simulink model "implementation"  (R2014b)
settings: Solver=ode45  StartTime=0.0  StopTime=4  RelTol=1e-3
values from neighbouring files (symbols this model uses):
  DEN = DEN{1}(2:end)    [print_control.m]
  dv = 1e-5    (= 1e-05)    [DCparamsPD.m]    (also in DCparamsPI.m; DCparamsPID.m)
  eta = 0.74    [DCparamsPD.m]    (also in DCparamsPI.m = 0.75; DCparamsPID.m = 0.75)
  J = 0.05    [DCparamsPD.m]    (also in DCparamsPI.m; DCparamsPID.m; beam_friction.m = 0.000914666666667)
  K = 0.0229    [DCparamsPD.m]    (also in DCparamsPI.m = 0.0214; DCparamsPID.m = 0.0214)
  k_f = [0.072091, 0.040963, -0.003493]    [DCparamsPD.m]    (also in DCparamsPI.m; DCparamsPID.m)
  L = 0.192e-3    (= 0.000192)    [DCparamsPD.m]    (also in DCparamsPI.m = 0.000129; DCparamsPID.m = 0.000129; beam_friction.m = 0.2)
  n = 300564.0/1300.0    (= 231.203076923)    [DCparamsPD.m]    (also in DCparamsPI.m = 149.526172053; DCparamsPID.m = 149.526172053; print_control.m = %0.4f)
  NUMfb = NUMfb{1}    [print_control.m]
  NUMff = NUMff{1}    [print_control.m]
  R = 1.83 + 0.33    (= 2.16)    [DCparamsPD.m]    (also in DCparamsPI.m = 1.07; DCparamsPID.m = 1.07; furuta_controller.m = 10; ik_test.m = 0.15925)
  Ts = 1 / 320    (= 0.003125)    [DCparamsPD.m]    (also in DCparamsPI.m = 0.002; DCparamsPID.m = 0.0016; ik_test.m = 0.0333333333333; read_log_file.m = mean(diff(D{end}.time)))
libraries: cstblocks x2, simulink x1
settings Model: Creator=vkozma  LastModifiedBy=vkozma

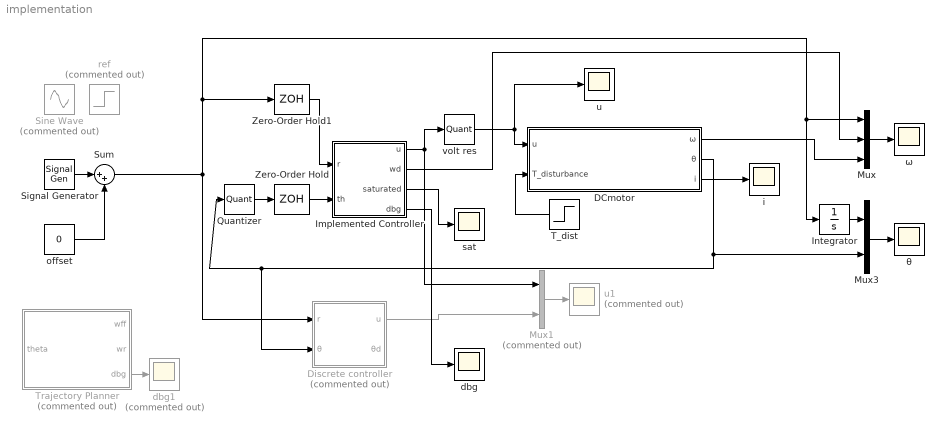
== system implementation ==
  DCmotor : Subsystem
  Discrete controller : Subsystem  Commented=on
  Implemented Controller : MATLAB Function  TreatAsAtomicUnit=on
  Integrator : Integrator
  Mux : Mux  Inputs=3
  Mux1 : Mux  Commented=on  Inputs=2
  Mux3 : Mux  Inputs=2
  Quantizer : Quantizer  QuantizationInterval=enc_res
  Signal Generator : SignalGenerator  WaveForm=square  Amplitude=2
  Sine Wave : Sin  Commented=on  Amplitude=2  Frequency=2*pi/4  SampleTime=0
  Sum : Sum  Inputs=|++
  T_dist : Step  Time=2  After=0  SampleTime=0
  Trajectory Planner : MATLAB Function  Commented=on  TreatAsAtomicUnit=on
  Zero-Order Hold : ZeroOrderHold  SampleTime=Ts
  Zero-Order Hold1 : ZeroOrderHold  SampleTime=Ts
  dbg : Scope
      settings: SaveName=ScopeData9
  dbg1 : Scope  Commented=on
      settings: TimeRange=0.1147540983606558  YMin=-1  YMax=1  SaveName=ScopeData10
  i : Scope
      settings: SaveName=ScopeData2
  offset : Constant  Value=0
  ref : Step  Commented=on  Time=0  After=-2  SampleTime=0
  sat : Scope
      settings: SaveName=ScopeData4
  u : Scope
  u1 : Scope  Commented=on
      settings: SaveName=ScopeData3
  volt res : Quantizer  QuantizationInterval=volt_res
  θ : Scope
      settings: SaveName=ScopeData6
  ω : Scope
  wires:
  DCmotor/1(ω) -> Mux/3
  Mux/1 -> ω/1
  Implemented Controller/1(u) -> Mux1/1, volt res/1
  DCmotor/2(θ) -> Mux3/2, Discrete controller/2(θ), Quantizer/1
  Implemented Controller/2(wd) -> Mux/2
  DCmotor/3(i) -> i/1
  T_dist/1 -> DCmotor/2(T_disturbance)
  Quantizer/1 -> Zero-Order Hold/1
  Zero-Order Hold/1 -> Implemented Controller/2(th)
  Zero-Order Hold1/1 -> Implemented Controller/1(r)
  Mux1/1 -> u1/1
  Discrete controller/1(u) -> Mux1/2
  Mux3/1 -> θ/1
  Implemented Controller/3(saturated) -> sat/1
  Implemented Controller/4(dbg) -> dbg/1
  Signal Generator/1 -> Sum/1
  offset/1 -> Sum/2
  Integrator/1 -> Mux3/1
  Sum/1 -> Zero-Order Hold1/1, Mux/1, Integrator/1, Discrete controller/1(r)
  volt res/1 -> DCmotor/1(u), u/1
  Trajectory Planner/3(dbg) -> dbg1/1

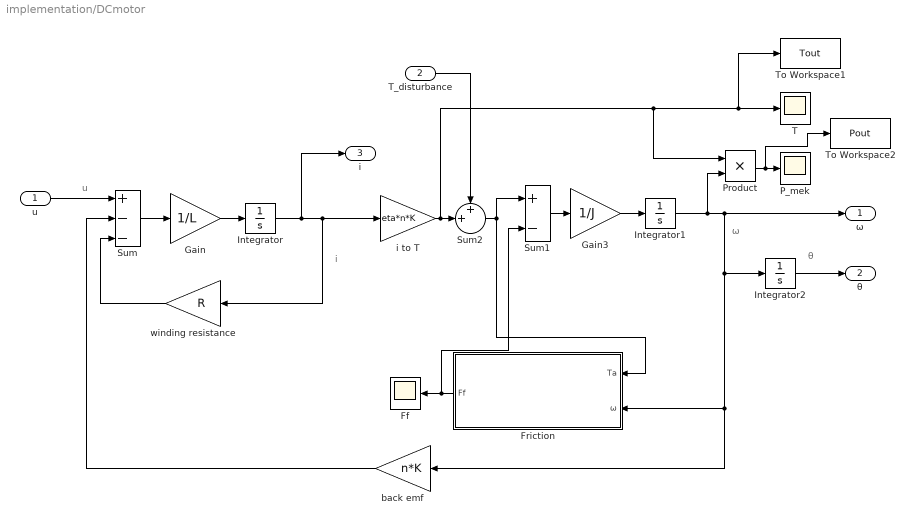
== system implementation/DCmotor ==
  note: θ
  note: ω
  note: i
  note: u
  u : Inport
  T_disturbance : Inport  Port=2
  Ff : Scope
      settings: SaveName=ScopeData5
  Friction : Subsystem
  Gain : Gain  Gain=1/L
  Gain3 : Gain  Gain=1/J
  Integrator : Integrator
  Integrator1 : Integrator
  Integrator2 : Integrator
  P_mek : Scope
      settings: SaveName=ScopeData8
  Product : Product
  Sum : Sum  Inputs=+--
  Sum1 : Sum  Inputs=+-
  Sum2 : Sum  Inputs=++|
  T : Scope
      settings: SaveName=ScopeData7
  To Workspace1 : ToWorkspace  VariableName=Tout  SampleTime=1/100
      settings: Save2DSignal=2-D array (concatenate along first dimension)
  To Workspace2 : ToWorkspace  VariableName=Pout  SampleTime=1/100
      settings: Save2DSignal=2-D array (concatenate along first dimension)
  back emf : Gain  Gain=n*K
  i to T : Gain  Gain=eta*n*K
  winding resistance : Gain  Gain=R
  ω : Outport
  θ : Outport  Port=2
  i : Outport  Port=3
  wires:
  u/1 -> Sum/1
  Sum/1 -> Gain/1
  Gain/1 -> Integrator/1
  Integrator/1 -> i/1, winding resistance/1, i to T/1
  winding resistance/1 -> Sum/3
  Sum1/1 -> Gain3/1
  Gain3/1 -> Integrator1/1
  Integrator1/1 -> Product/2, ω/1, Integrator2/1, Friction/2(ω), back emf/1
  i to T/1 -> Sum2/2, Product/1, To Workspace1/1, T/1
  back emf/1 -> Sum/2
  Integrator2/1 -> θ/1
  Product/1 -> To Workspace2/1, P_mek/1
  Friction/1(Ff) -> Sum1/2, Ff/1
  Sum2/1 -> Friction/1(Ta), Sum1/1
  T_disturbance/1 -> Sum2/1

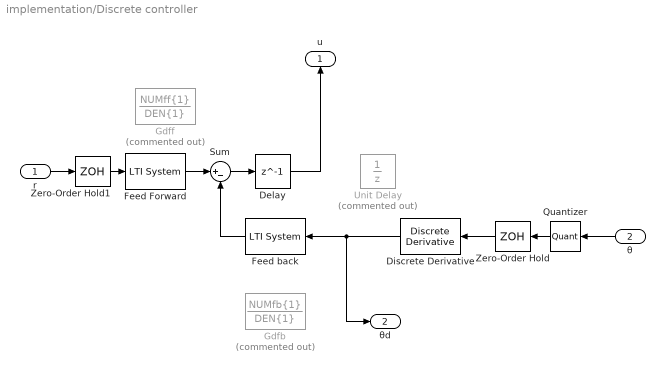
== system implementation/Discrete controller ==
  r : Inport
  θ : Inport  Port=2
  Delay : Delay  DelayLength=1
  Discrete Derivative : simulink/Discrete/Discrete Derivative  gainval=1.0  ICPrevScaledInput=0.0  InputProcessing=Inherited  OutMin=[]  OutMax=[]  OutDataType=fixdt(1, 16)  OutScaling=2^-10  DoSatur=off
  Feed Forward : cstblocks/LTI System  sys=Gdff  IC=[]
  Feed back : cstblocks/LTI System  sys=Gdfb  IC=[]
  Gdfb : DiscreteTransferFcn  Commented=on  Numerator=NUMfb{1}  Denominator=DEN{1}
  Gdff : DiscreteTransferFcn  Commented=on  Numerator=NUMff{1}  Denominator=DEN{1}
  Quantizer : Quantizer  QuantizationInterval=enc_res
  Sum : Sum  Inputs=|+-
  Unit Delay : UnitDelay  Commented=on  SampleTime=-1
  Zero-Order Hold : ZeroOrderHold  SampleTime=Ts
  Zero-Order Hold1 : ZeroOrderHold  SampleTime=Ts
  u : Outport
  θd : Outport  Port=2
  wires:
  r/1 -> Zero-Order Hold1/1
  θ/1 -> Quantizer/1
  Quantizer/1 -> Zero-Order Hold/1
  Zero-Order Hold/1 -> Discrete Derivative/1
  Sum/1 -> Delay/1
  Discrete Derivative/1 -> Feed back/1, θd/1
  Zero-Order Hold1/1 -> Feed Forward/1
  Delay/1 -> u/1
  Feed back/1 -> Sum/2
  Feed Forward/1 -> Sum/1

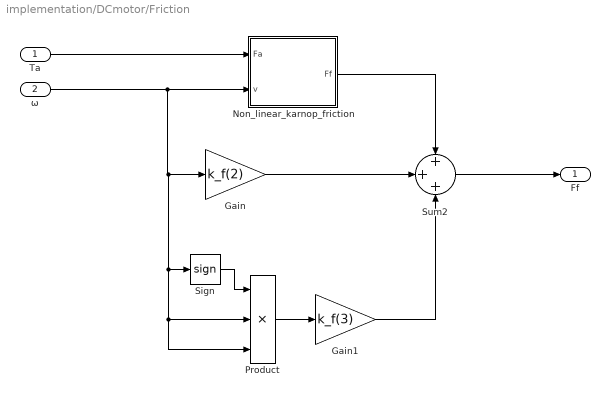
== system implementation/DCmotor/Friction ==
  Ta : Inport
  ω : Inport  Port=2
  Gain : Gain  Gain=k_f(2)
  Gain1 : Gain  Gain=k_f(3)
  Non_linear_karnop_friction : Subsystem
  Product : Product  Inputs=3
  Sign : Signum
  Sum2 : Sum  Inputs=+++
  Ff : Outport
  wires:
  ω/1 -> Product/3, Product/2, Sign/1, Gain/1, Non_linear_karnop_friction/2(v)
  Ta/1 -> Non_linear_karnop_friction/1(Fa)
  Sum2/1 -> Ff/1
  Non_linear_karnop_friction/1(Ff) -> Sum2/1
  Gain/1 -> Sum2/2
  Sign/1 -> Product/1
  Product/1 -> Gain1/1
  Gain1/1 -> Sum2/3

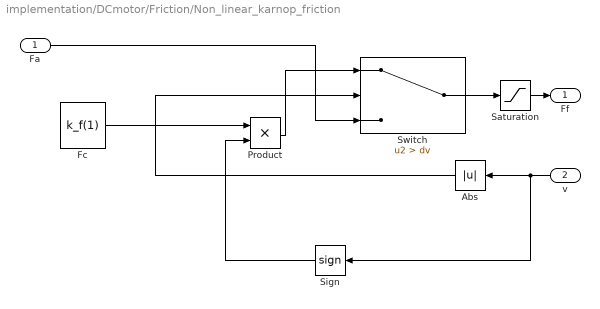
== system implementation/DCmotor/Friction/Non_linear_karnop_friction ==
  Fa : Inport
  v : Inport  Port=2
  Abs : Abs
  Fc : Constant  Value=k_f(1)
  Product : Product  RndMeth=Zero
  Saturation : Saturate  UpperLimit=k_f(1)  LowerLimit=-k_f(1)
  Sign : Signum
  Switch : Switch  Criteria=u2 > Threshold  Threshold=dv
  Ff : Outport
  wires:
  Sign/1 -> Product/2
  Fc/1 -> Product/1
  Abs/1 -> Switch/2
  Fa/1 -> Switch/3
  v/1 -> Abs/1, Sign/1
  Switch/1 -> Saturation/1
  Saturation/1 -> Ff/1
  Product/1 -> Switch/1

== matlab function implementation/Trajectory Planner ==
  data: wff output; theta input; wr output; dbg output
function [wff,wr,dbg] = fcn(theta)
% Trajectory planning for a speed controller
persistent theta_goal w_ff state theta_tot T_on prev_err cum_err dbg_val
persistent w_acc w_trans Ts P I D % Constants
if isempty(w_ff) % init traj planner
    % Inputs and stuff that may change
    theta_goal = 3;
    w_ff = 0;
    state = 3; % 0 = acc to w_trans, 1 = steady speed, 2 = decelerate to 0, 3 = keep at 0
    theta_tot = 0;
    T_on = 0; % timer
    prev_err = 0; cum_err = 0; % Feedback control
    dbg_val = 1;
    % Constants
    w_acc = 5; % rad/s/s
    w_trans = 1.8377; % rad/s
    Ts = 1/500; % Sample time
    P = 12.925; I = 37.0; D = 0.3; % PID-constants 
end % init

%%%%%%%%%%%%%%%%%%%%%%%%%% MASTER UNIT %%%%%%%%%%%%%%%%%%%%%%%%%%%%%%%%%

% Master unit, for issuing commands
persistent Ts_master prev_time pressed
if isempty(Ts_master) % init master
    Ts_master = 1/50;
    prev_time = 0;
    pressed = 0;
end
% Master loop
if (T_on - prev_time >= Ts_master)
    if pressed == 0 && T_on >= 2.5
        pressed = 1;
        theta_goal = 4;
        w_trans = 3.618033;
    end
    
    prev_time = T_on;%prev_time + Ts_master;
end

%%%%%%%%%%%%%%%%%%%%%% TRAJECTORY PLANNER %%%%%%%%%%%%%%%%%%%%%%%%%%%%%

% Check whether to start to break 
if (state < 2) && (abs(theta_goal - theta_tot) < w_ff*w_ff/(2*w_acc))
    state = 2;
end

switch state
    case 0 % acc to w_trans
        new_w = w_ff + sign(sign(theta_goal+eps)*w_trans - w_ff)*Ts*w_acc;
        if sign(new_w - sign(theta_goal+eps)*w_trans + eps) ~= sign(w_ff - sign(theta_goal+eps)*w_trans + eps)
            w_ff = sign(theta_goal+eps)*w_trans;
            state = 1;
        else
            w_ff = new_w;
        end
        
    case 1 % steady speed
        if abs(w_ff - sign(theta_goal+eps)*w_trans) > 1e-6 % new speed found
            state = 0;
        else
            w_ff = sign(theta_goal+eps)*w_trans;
        end
    case 2 % decelerate to zero speed
        new_w = w_ff - sign(w_ff+eps)*Ts*w_acc;
        if sign(new_w) ~= sign(w_ff)
            w_ff = 0;
            state = 3;
        else
            w_ff = new_w;
        end
    case 3 % stay at zero, at target
        w_ff = 0;
        if abs(theta_tot - theta_goal) < 1e-2
            theta_tot = theta_goal;
        end
        if abs(theta_tot - theta_goal) > 1e-3;
            state = 0;
            fprintf('t = %f, theta_tot = %f, theta_goal = %f\n',T_on,theta_tot,theta_goal);
        end
end

% feedback PID-control
err = theta_tot - theta;
w_fb = P*err + I*cum_err + D*(err - prev_err)/Ts;
prev_err = err;
cum_err = cum_err + err*Ts;

% Output 
wr = w_ff + w_fb;
wff = w_ff;

% debugging var
dbg = dbg_val;

% Update theta_tot
theta_tot = theta_tot + Ts * w_ff;
T_on = T_on + Ts;
end

== matlab function implementation/Implemented Controller ==
  data: r input; th input; u output; wd output; saturated output; dbg output
function [u,wd,saturated,dbg] = fcn(r,th)
persistent uout old_y old_r old_uff old_ufb prev_th I_ff I_fb old_spd issat
persistent cMode Ts nd d nc c nf f Id umax imax K R n% Constants
if isempty(uout) % init
    uout = 0; issat = 0;
    old_y = zeros(1,4); old_r = zeros(1,4);
    old_uff = zeros(1,4); old_ufb = zeros(1,4);
    prev_th = 0; I_ff = 0; I_fb = 0;
    old_spd = 0;
    % Generated constants from script, replace if new params
K = 0.0214; n = 149.5262; R = 1.0700;
cMode = 1; umax = 24.0; imax = 2.0;
Ts = 1/500.00;
nd = 2; d = [0.02358463,0.02358463];
nc = 2; c = [-0.62039556,0.88517879];
nf = 1; f = [-0.68842077];
Id = 0.20189841;
end % of init
u = uout;

if cMode == 0
    old_y(1) = th; %wd = (th - prev_th)/Ts; % Position control
else
    old_y(1) = (th - prev_th)/Ts; %wd = old_y(1); % Speed control
end
old_r(1) = r;

% ufb = d(2)*old_y(1) + d(1)*old_y(2) - f(2)*old_ufb(1) - f(1)*old_ufb(2);
% uff = c(3)*old_r(1) + c(2)*old_r(2) + c(1)*old_r(3) - f(2)*old_uff(1) - f(1)*old_uff(2);
ufb = 0; uff = 0;
for i = 1:nd
    ufb = ufb + d(i)*old_y(nd-i+1);
end
for i = 1:nc
    uff = uff + c(i)*old_r(nc-i+1);
end
for i = 1:nf
    ufb = ufb - f(i)*old_ufb(nf-i+1);
    uff = uff - f(i)*old_uff(nf-i+1);
end

% Integrators
skipping = 0.99;
%T_backcalc = 0.05;
if Id > 0 && issat == 0
%if Id > 0 && issat == 0 && (old_r(1) - old_y(1))*u_nosat >= 0
%if Id > 0 && issat == 0 && (I_ff - I_fb)*u_nosat >= 0
%if Id > 0
%     I_ff = I_ff + (Id + Ts*(uout - u_nosat)/T_backcalc)*old_r(1);
%     I_fb = I_fb + (Id - Ts*(uout - u_nosat)/T_backcalc)*old_y(1);
    I_ff = I_ff + Id*old_r(1);
    I_fb = I_fb + Id*old_y(1);
    skipping = 0.01;
end

% if Id > 0 % Skip if no integrator term is present
%     toupdate = 1;
%     if issat == 1 % if saturated don't update the terms
%         if sign(I_ff - I_fb) ~= sign(u_nosat) % if can't reach
%             toupdate = 0;
%         end
%         toupdate = 0;
%     end
%     if toupdate == 1
%         I_ff = I_ff + Id*old_r(1);
%         I_fb = I_fb + Id*old_y(1);
%         skipping = 0.01; % debug variable
%     end
% end


saturated = 0.98*issat + 0.01; % test

uout = (uff + I_ff) - (ufb + I_fb);

% Current and voltage limiting
issat = 0; u_nosat = uout;
% voltage limiting
if uout > umax
    uout = umax;
    issat = 1;
elseif uout < -umax
    uout = -umax;
    issat = 1;
end

% current limiting
%if Id == 0 % Anti windup may get wonky with the current limiter
    curr_lim_dlpfc = 0.2;
    spd = (th - prev_th)/Ts;
    spd = curr_lim_dlpfc*spd + (1 - curr_lim_dlpfc)*old_spd;
    old_spd = spd;
    temp1 = K*n*spd; temp2 = R*imax;
    if uout > (temp1 + temp2), 
        uout = temp1 + temp2; 
        issat = 1;
    elseif uout < (temp1 - temp2) 
        uout = temp1 - temp2; 
        issat = 1;
    end
%end

% Debugging output
wd = (th - prev_th)/Ts; 
dbg = [skipping,saturated];%, 1.01*sign(I_ff - I_fb), 0.95*sign(old_r(1) - old_y(1))]; %[uff - ufb, I_ff - I_fb];

% % To counter floating point rounding errors
% if max(abs(I_ff),abs(I_fb)) > 100 
%     I_fb = I_fb - I_ff;
%     I_ff = 0;
% end

% Update old values
for i = 3:-1:1
    old_y(i+1) = old_y(i); old_r(i+1) = old_r(i);
    old_uff(i+1) = old_uff(i); old_ufb(i+1) = old_ufb(i);
end
old_ufb(1) = ufb; old_uff(1) = uff;
prev_th = th;
%fprintf('old_uff = [%f, %f, %f, %f]\n',old_uff(1),old_uff(2),old_uff(3),old_uff(4));

end
